simulink model "phaser (1)"  (R2024a)
settings: Solver=VariableStepAuto  StartTime=0.0  StopTime=120  RelTol=1e-3
values from neighbouring files (symbols this model uses):
  c = (tan(pi*BW/fs)-1)/(tan(pi*BW/fs)+1)    [II_order_allpass_IIR.m]
  d = -cos(2*pi*fb/fs)    [II_order_allpass_IIR.m]
libraries: dspsnks4 x1, dspvision x1
settings Model: Creator=EAGLEAORUS  LastModifiedBy=EAGLEAORUS

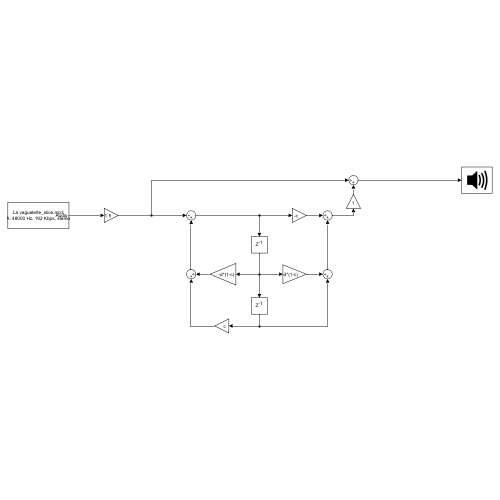
[thumbnail: Simulink's stored preview of the top-level diagram]
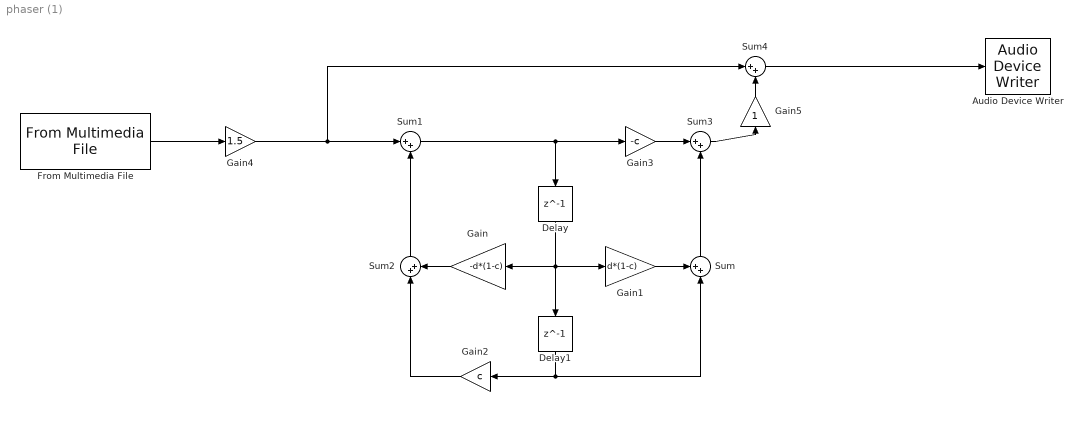
== system phaser (1) ==
  Audio Device Writer : dspsnks4/Audio Device Writer  Driver=DirectSound  Device=Default  InheritSampleRate=on  SampleRate=44100  BitDepth=16-bit integer  BufferSize=4096  NumBuffers=10  DefaultOutputChannelMapping=on  OutputChannelMapping=1:2  OutputNumUnderrunSamples=off  DriverIdx=1  DeviceWarnFlag=''
  Delay : Delay  DelayLength=1  InitialCondition=0
  Delay1 : Delay  DelayLength=1  InitialCondition=0
  From Multimedia File : dspvision/From Multimedia File  inputFilename=C:\Users\EAGLEAORUS\Desktop\playing_FPGA\自制音频片段\La vaguelette_slice.mp3  readRange=[1 Inf]  loop=on  numPlays=inf  outputStreams=Audio only  videoDataType=single  audioDataType=double  inheritSampleTime=on  userDefinedSampleTime=1/30  noAudioOutput=off  isIntensityVideo=off  fourcc=RGB  colorVideoFormat=Separate color signals  outputEOF=off  dataOrg=Column-major  audioFrameSize=1024  computeAudioFrameSize=off  outSamplingMode=Sample based
      settings: LibrarySourceBlock=audiosources/From Multimedia File
  Gain : Gain  Gain=-d*(1-c)
  Gain1 : Gain  Gain=d*(1-c)
  Gain2 : Gain  Gain=c
  Gain3 : Gain  Gain=-c
  Gain4 : Gain  Gain=1.5
  Gain5 : Gain
  Sum : Sum  Inputs=++|
  Sum{1..4} (4 alike) : Sum  Inputs=|++
  wires:
  Gain2/1 -> Sum2/1
  Delay1/1 -> Sum/2, Gain2/1
  Sum/1 -> Sum3/2
  Sum1/1 -> Gain3/1, Delay/1
  Gain3/1 -> Sum3/1
  From Multimedia File/1 -> Gain4/1
  Gain/1 -> Sum2/2
  Sum2/1 -> Sum1/2
  Delay/1 -> Delay1/1, Gain/1, Gain1/1
  Gain1/1 -> Sum/1
  Sum3/1 -> Gain5/1
  Gain5/1 -> Sum4/2
  Sum4/1 -> Audio Device Writer/1
  Gain4/1 -> Sum4/1, Sum1/1
